simulink model "inverter"  (R2015a)
settings: Solver=ode45  StartTime=0.0  StopTime=1000  RelTol=1e-3
libraries: powerlib x13, powerlib_meascontrol x1
settings Model: Creator=Kelvin Gakuo  LastModifiedBy=Kelvin Gakuo

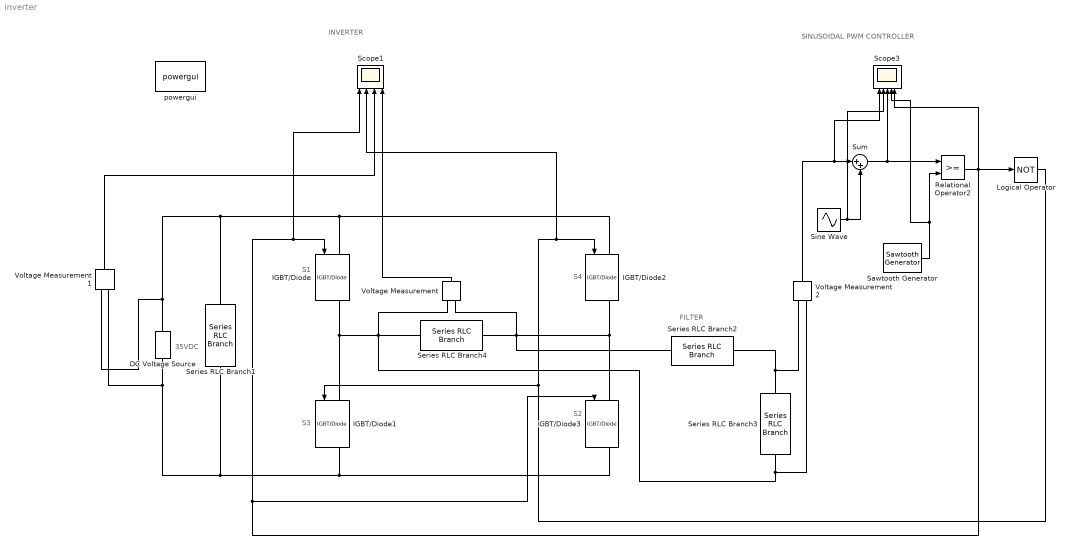
== system inverter ==
  note: 35VDC
  note: S3
  note: S4
  note: S2
  note: S1
  note: SINUSOIDAL PWM CONTROLLER
  note: INVERTER
  note: FILTER
  DC Voltage Source : powerlib/Electrical Sources/DC Voltage Source  Amplitude=35  Measurements=None
  IGBT/Diode{,1..3} (4 alike) : powerlib/Power Electronics/IGBT//Diode  Ron=1e-3  Rs=1e5  Cs=inf  Measurements=on
  Logical Operator : Logic  Operator=NOT  AllPortsSameDT=off  OutDataTypeStr=boolean
  Relational Operator2 : RelationalOperator  OutDataTypeStr=boolean  ZeroCross=off
  Sawtooth Generator : powerlib_meascontrol/Pulse & Signal Generators/Sawtooth Generator  Freq=80  Phase=180  Ts=0
  Scope1 : Scope  NumInputPorts=4
      settings: TimeRange=0.1  YMin=-0.2~-0.2~35~-40  YMax=1.2~1.2~35~40
  Scope3 : Scope  NumInputPorts=5
      settings: TimeRange=0.1  YMin=-1.5~-1~-2~-1~-0.2  YMax=1.5~1~2~1~1.2  SaveName=ScopeData2
  Series RLC Branch1 : powerlib/Elements/Series RLC Branch  LConnTagsString=__new0  RConnTagsString=__new0  BranchType=RC  Resistance=1  Inductance=1e-3  SetiL0=off  InitialCurrent=0  Capacitance=0.7e-3  Setx0=off  InitialVoltage=0  Measurements=None
  Series RLC Branch2 : powerlib/Elements/Series RLC Branch  LConnTagsString=__new0  RConnTagsString=__new0  BranchType=RL  Resistance=100  Inductance=120e-3  SetiL0=off  InitialCurrent=0  Capacitance=0.7e-3  Setx0=off  InitialVoltage=0  Measurements=None
  Series RLC Branch3 : powerlib/Elements/Series RLC Branch  LConnTagsString=__new0  RConnTagsString=__new0  BranchType=C  Resistance=100  Inductance=120e-3  SetiL0=off  InitialCurrent=0  Capacitance=0.7e-3  Setx0=off  InitialVoltage=0  Measurements=None
  Series RLC Branch4 : powerlib/Elements/Series RLC Branch  LConnTagsString=__new0  RConnTagsString=__new0  BranchType=R  Resistance=100  Inductance=120e-3  SetiL0=off  InitialCurrent=0  Capacitance=0.7e-3  Setx0=off  InitialVoltage=0  Measurements=None
  Sine Wave : Sin  Frequency=2*pi*80  SampleTime=0
  Sum : Sum  Inputs=|++
  Voltage Measurement : powerlib/Measurements/Voltage Measurement  PhasorSimulation=off  OutputType=Complex  PSBequivalent=0
  Voltage Measurement1 : powerlib/Measurements/Voltage Measurement  PhasorSimulation=off  OutputType=Complex  PSBequivalent=0
  Voltage Measurement2 : powerlib/Measurements/Voltage Measurement  PhasorSimulation=off  OutputType=Complex  PSBequivalent=0
  powergui : powerlib/powergui  Priority=1  SimulationMode=Discrete  SolverType=Tustin/Backward Euler (TBE)  SampleTime=50e-6  frequency=60  SPID=off  DisableSnubberDevices=off  DisableRonSwitches=off  DisableVfSwitches=off  SwTol=0  DisplayEquations=off  Interpol=off  methode=off  Ts=100  FunctionMessages=off  echomessages=off  HookPort=off  EnableUseOfTLC=off  x0status=blocks  frequencyindice=0  Pbase=100e6  ErrMax=1e-4  Iterations=50  UnitsV=kV  UnitsW=MW  buscounter=0  RestoreLinks=warning  ResistiveCurrentMeasurement=off  Frange=[0:2:500]  Ylog=off  Xlog=on  ShowGrid=off  save=off  variable=ZData  structure=0  ZoomFFT=off  StartTime=0.0  cycles=1  DisplayStyle=1  fundamental=60  FreqAxis=off  MaxFrequency=1000  frequencyindicesteady=1  RmsSteady=1  display=off
  wires:
  Voltage Measurement1/1 -> Scope1/3
  Voltage Measurement/1 -> Scope1/4
  Voltage Measurement2/1 -> Scope3/1, Sum/1
  Sine Wave/1 -> Sum/2, Scope3/2
  Sum/1 -> Relational Operator2/1, Scope3/3
  Sawtooth Generator/1 -> Scope3/4, Relational Operator2/2
  Relational Operator2/1 -> IGBT/Diode/1, Scope1/1, IGBT/Diode3/1, Logical Operator/1, Scope3/5
  Logical Operator/1 -> IGBT/Diode2/1, Scope1/2, IGBT/Diode1/1
  connections:
  DC Voltage Source/RConn1 -- Voltage Measurement1/LConn1 -- Series RLC Branch1/RConn1 -- IGBT/Diode/LConn1 -- IGBT/Diode2/LConn1
  DC Voltage Source/LConn1 -- Voltage Measurement1/LConn2 -- Series RLC Branch1/LConn1 -- IGBT/Diode1/RConn1 -- IGBT/Diode3/RConn1
  IGBT/Diode3/LConn1 -- Series RLC Branch2/RConn1 -- Voltage Measurement/LConn2 -- Series RLC Branch4/RConn1 -- IGBT/Diode2/RConn1
  Voltage Measurement/LConn1 -- Voltage Measurement2/LConn2 -- Series RLC Branch3/RConn1 -- Series RLC Branch4/LConn1 -- IGBT/Diode/RConn1 -- IGBT/Diode1/LConn1
  Series RLC Branch2/LConn1 -- Voltage Measurement2/LConn1 -- Series RLC Branch3/LConn1
